simulink library "PID_continous_block"  (Simulink 2.20)

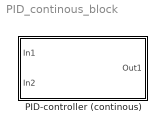
== system PID_continous_block ==
  PID-controller (continous) : Subsystem  Description=PID_regulator  mask{P=1, I=25, D=1}
      mask prompts: P "P="; I "I="; D "D="
      mask help: PID continous controller
      mask init:
      | q0=P;
      | q1=P/I;
      | q2=P*D;
      mask Help: Enter P,I,D,T

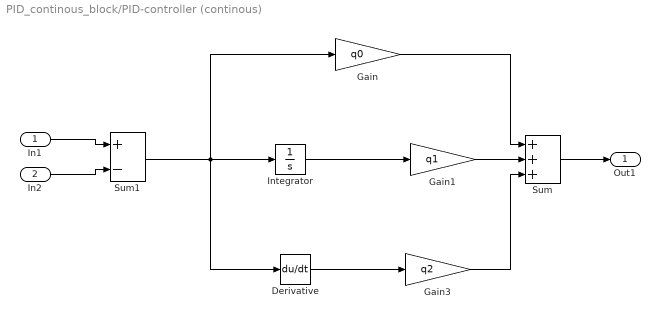
== system PID_continous_block/PID-controller (continous) ==
  In1 : Inport  Port=1  PortWidth=-1  SampleTime=-1
  In2 : Inport  Port=2  PortWidth=-1  SampleTime=-1
  Derivative : Derivative
  Gain : Gain  Gain=q0
  Gain1 : Gain  Gain=q1
  Gain3 : Gain  Gain=q2
  Integrator : Integrator  ExternalReset=none  InitialConditionSource=internal  InitialCondition=0  LimitOutput=off  UpperSaturationLimit=inf  LowerSaturationLimit=-inf  ShowSaturationPort=off  ShowStatePort=off  AbsoluteTolerance=auto
  Sum : Sum  Inputs=+++
  Sum1 : Sum  Inputs=+-
  Out1 : Outport  Port=1
  wires:
  In2/1 -> Sum1/2
  In1/1 -> Sum1/1
  Sum1/1 -> Gain/1, Integrator/1, Derivative/1
  Gain/1 -> Sum/1
  Gain1/1 -> Sum/2
  Integrator/1 -> Gain1/1
  Sum/1 -> Out1/1
  Gain3/1 -> Sum/3
  Derivative/1 -> Gain3/1
